simulink model "AC_DC_Converter_SEDC_Motor"  (R2023a)
settings: Solver=VariableStepAuto  StartTime=0.0  StopTime=10  MaxStep=0.001  RelTol=1e-3
libraries: spsThyristorLib x4, spsVoltageMeasurementLib x3, spsSeriesRLCBranchLib x2, simulink x2, dspswit3 x1, spsUniversalBridgeLib x1, spsACVoltageSourceLib x1, sps_lib x1
settings Model: Creator=Mohamed Ezzelrgal  LastModifiedBy=Mohamed Ezzelrgal

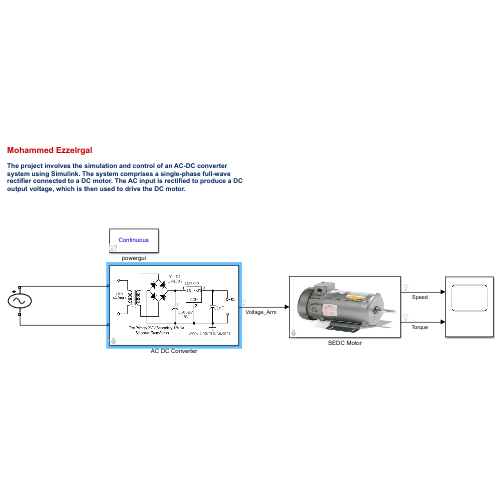
[thumbnail: Simulink's stored preview of the top-level diagram]
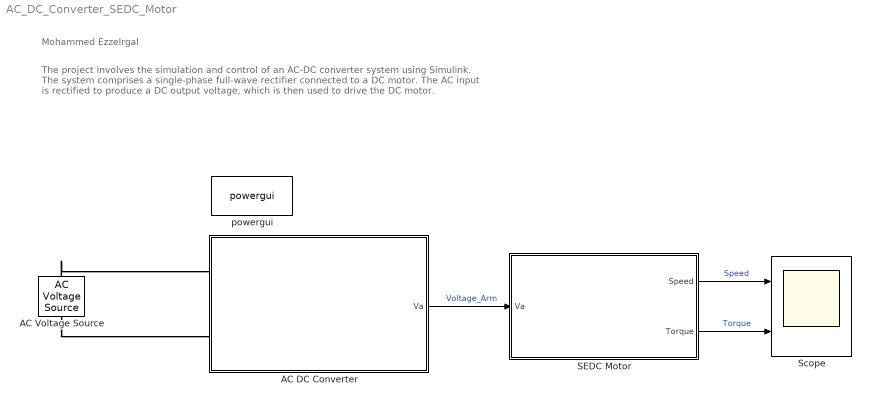
== system AC_DC_Converter_SEDC_Motor ==
  note: Mohammed Ezzelrgal
  note: The project involves the simulation and control of an AC-DC converter system using Simulink. The system comprises a single-phase full-wave rectifier connected to a DC motor. The AC input is rectified to produce a DC output voltage, which is then used to drive the DC motor.
  AC DC Converter : Subsystem  mask{Firing_Angle=20}
      mask prompts: Firing_Angle "Firing Angle"
      mask DialogControl DescGroupVar Prompt: AC-DC Converter
      mask DialogControl DescTextVar Prompt: This conversion process involves changing the polarity of the input AC voltage to produce a unidirectional flow of current in the output DC circuit. AC-DC converters are essential components in various electronic devices and power supplies, allowing them to operate using DC power from an AC power source.
      mask Display: image('acdc.png');
  AC Voltage Source : spsACVoltageSourceLib/AC Voltage Source  Amplitude=sqrt(2)*20  Phase=0  Frequency=50  SampleTime=0  Measurements=None  BusType=swing  Pref=10e3  Qref=0  Qmin=-inf  Qmax=+inf
  SEDC Motor : Subsystem  mask{La=0.1, K_phi=1.6, TL=20, Ra=0.5, J=5, B=0.01}
      mask prompts: K_phi "K Phi"; TL "Torqu Load"
      mask DialogControl DescGroupVar Prompt: SEDC Motor
      mask DialogControl DescTextVar Prompt: Modeling a separately excited DC motor in Simulink involves representing the electrical and mechanical components of the  motor system
      mask Display: image('SEDC.png');
  Scope : Scope  NumInputPorts=2
  powergui : sps_lib/powergui  Priority=1  SimulationMode=Continuous  SampleTime=50e-6  frequency=60  Iterations=50  frequencyindice=50  Pbase=100e6  ErrMax=1e-4  UnitsV=kV  UnitsW=MW  buscounter=0  FunctionMessages=off  echomessages=off  EnableUseOfTLC=off  CurrentSourceSwitches=off  DisableSnubberDevices=off  DisableRonSwitches=off  DisableVfSwitches=off  DisplayEquations=off  AutomaticDiscreteSolvers=off  SolverType=Tustin/Backward Euler (TBE)  Interpol=off  ExternalGateDelay=off  methode=off  Ts=100  x0status=blocks  SPID=on  SwTol=0  HookPort=off  NonlinearTolerance=1e-4  nMaxIteration=100  ContinueOnMaxIteration=off  RestoreLinks=warning  ResistiveCurrentMeasurement=off  Frange=[0:2:500]  Ylog=off  Xlog=on  ShowGrid=off  save=off  variable=ZData  structure=0  ZoomFFT=off  StartTime=0.0  cycles=1  DisplayStyle=1  fundamental=60  FreqAxis=off  MaxFrequency=1000  frequencyindicesteady=1  RmsSteady=1  display=off
  wires:
  SEDC Motor/2(Torque) -> Scope/2  "Torque"
  SEDC Motor/1(Speed) -> Scope/1  "Speed"
  AC DC Converter/1(Va) -> SEDC Motor/1(Va)  "Voltage_Arm"
  connections:
  AC Voltage Source/RConn1 -- AC DC Converter/LConn1
  AC Voltage Source/LConn1 -- AC DC Converter/LConn2

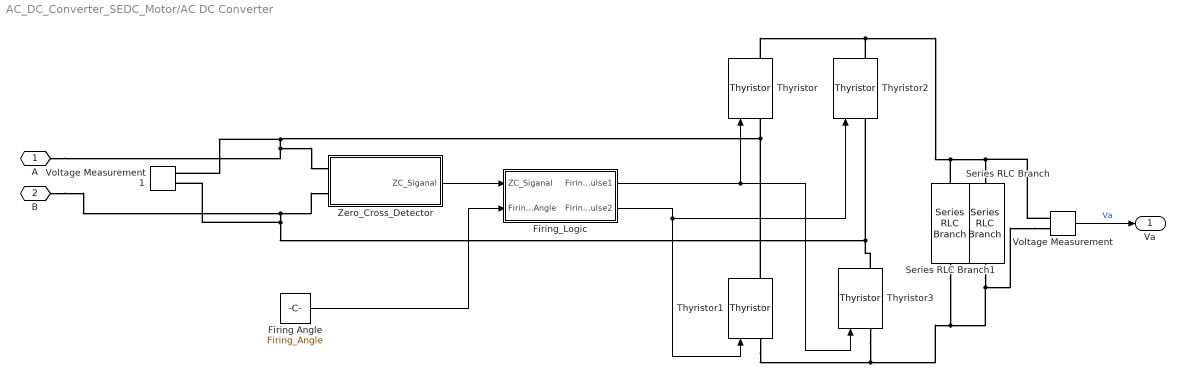
== system AC_DC_Converter_SEDC_Motor/AC DC Converter ==
  Firing Angle : Constant  Value=Firing_Angle
  Firing_Logic : Subsystem
  Series RLC Branch : spsSeriesRLCBranchLib/Series RLC Branch  LConnTagsString=__new0  RConnTagsString=__new0  BranchType=R  Resistance=50  Inductance=1e-3  SetiL0=off  InitialCurrent=0  Capacitance=1e-6  Setx0=off  InitialVoltage=0  Measurements=None
  Series RLC Branch1 : spsSeriesRLCBranchLib/Series RLC Branch  LConnTagsString=__new0  RConnTagsString=__new0  BranchType=C  Resistance=50  Inductance=1e-3  SetiL0=off  InitialCurrent=0  Capacitance=1  Setx0=off  InitialVoltage=0  Measurements=None
  Thyristor{,1..3} (4 alike) : spsThyristorLib/Thyristor  Ron=0.001  Lon=0  Vf=0.8  IC=0  Rs=500  Cs=250e-9  Measurements=on
  Voltage Measurement : spsVoltageMeasurementLib/Voltage Measurement  PhasorSimulation=off  OutputType=Complex  PSBequivalent=0
  Voltage Measurement1 : spsVoltageMeasurementLib/Voltage Measurement  PhasorSimulation=off  OutputType=Complex  PSBequivalent=0
  Zero_Cross_Detector : Subsystem
  A : PMIOPort  Side=Left
  B : PMIOPort  Port=2  Side=Left
  Va : Outport
  wires:
  Firing_Logic/1(Firing_Pulse1) -> Thyristor3/1, Thyristor/1
  Firing_Logic/2(Firing_Pulse2) -> Thyristor2/1, Thyristor1/1
  Zero_Cross_Detector/1(ZC_Siganal) -> Firing_Logic/1(ZC_Siganal)
  Firing Angle/1 -> Firing_Logic/2(Firing_Angle)
  Voltage Measurement/1 -> Va/1  "Va"
  connections:
  Voltage Measurement1/LConn1 -- Thyristor2/LConn1 -- Thyristor3/RConn1 -- B/RConn1 -- Zero_Cross_Detector/LConn2
  Voltage Measurement1/LConn2 -- Thyristor1/RConn1 -- Thyristor/LConn1 -- A/RConn1 -- Zero_Cross_Detector/LConn1
  Thyristor2/RConn1 -- Thyristor/RConn1 -- Series RLC Branch1/LConn1 -- Voltage Measurement/LConn1 -- Series RLC Branch/LConn1
  Voltage Measurement/LConn2 -- Series RLC Branch1/RConn1 -- Thyristor1/LConn1 -- Thyristor3/LConn1 -- Series RLC Branch/RConn1

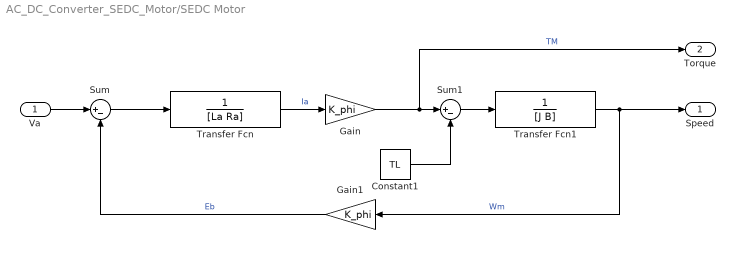
== system AC_DC_Converter_SEDC_Motor/SEDC Motor ==
  Va : Inport
  Constant1 : Constant  Value=TL
  Gain : Gain  Gain=K_phi
  Gain1 : Gain  Gain=K_phi
  Sum : Sum  Inputs=|+-
  Sum1 : Sum  Inputs=|+-
  Transfer Fcn : TransferFcn  Denominator=[La Ra]
  Transfer Fcn1 : TransferFcn  Denominator=[J B]
  Speed : Outport
  Torque : Outport  Port=2
  wires:
  Transfer Fcn/1 -> Gain/1  "Ia"
  Transfer Fcn1/1 -> Speed/1, Gain1/1  "Wm"
  Va/1 -> Sum/1
  Gain1/1 -> Sum/2  "Eb"
  Constant1/1 -> Sum1/2
  Sum/1 -> Transfer Fcn/1
  Gain/1 -> Torque/1, Sum1/1  "TM"
  Sum1/1 -> Transfer Fcn1/1

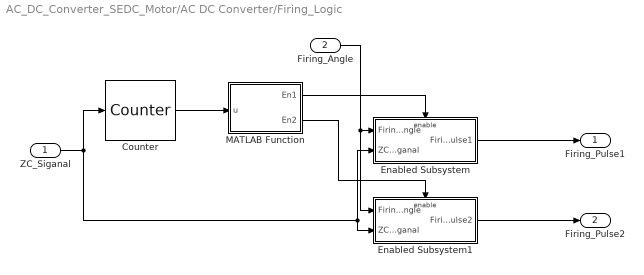
== system AC_DC_Converter_SEDC_Motor/AC DC Converter/Firing_Logic ==
  ZC_Siganal : Inport
  Firing_Angle : Inport  Port=2
  Counter : dspswit3/Counter  Direction=Up  CountEvent=Rising edge  CounterSize=User defined  MaxCount=255  InitialCount=0  Output=Count  HitValue=32  ResetInput=off  SamplesPerFrame=1  Ts=1  CntDtype=double  HitDtype=Logical
  Enabled Subsystem : Subsystem  TreatAsAtomicUnit=on
  Enabled Subsystem1 : Subsystem  TreatAsAtomicUnit=on
  MATLAB Function : MATLAB Function  TreatAsAtomicUnit=on
  Firing_Pulse1 : Outport
  Firing_Pulse2 : Outport  Port=2
  wires:
  ZC_Siganal/1 -> Enabled Subsystem/2(ZC_Siganal), Enabled Subsystem1/2(ZC_Siganal), Counter/1
  Counter/1 -> MATLAB Function/1(u)
  MATLAB Function/1(En1) -> Enabled Subsystem/Enable
  MATLAB Function/2(En2) -> Enabled Subsystem1/Enable
  Firing_Angle/1 -> Enabled Subsystem1/1(Firing_Angle), Enabled Subsystem/1(Firing_Angle)
  Enabled Subsystem/1(Firing_Pulse1) -> Firing_Pulse1/1
  Enabled Subsystem1/1(Firing_Pulse2) -> Firing_Pulse2/1

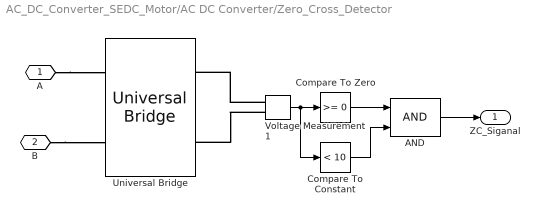
== system AC_DC_Converter_SEDC_Motor/AC DC Converter/Zero_Cross_Detector ==
  AND : Logic  IconShape=distinctive  AllPortsSameDT=off  OutDataTypeStr=boolean
  Compare To Constant : simulink/Logic and Bit Operations/Compare To Constant  relop=<  const=10  OutDataTypeStr=boolean
  Compare To Zero : simulink/Logic and Bit Operations/Compare To Zero  relop=>=  OutDataTypeStr=boolean
  Universal Bridge : spsUniversalBridgeLib/Universal Bridge  Arms=2  SnubberResistance=1e5  SnubberCapacitance=inf  Device=Diodes  Ron=1e-3  Lon=0  ForwardVoltages="[  0  0  ]"  ForwardVoltage=0  GTOparameters=[ 10e-6 , 20e-6 ]  IGBTparameters=[ 1e-6 , 2e-6 ]  Measurements=None  Measurements_2=None  converterType=Rectifier
  Voltage Measurement1 : spsVoltageMeasurementLib/Voltage Measurement  PhasorSimulation=off  OutputType=Complex  PSBequivalent=0
  A : PMIOPort  Side=Left
  B : PMIOPort  Port=2  Side=Left
  ZC_Siganal : Outport
  wires:
  Voltage Measurement1/1 -> Compare To Constant/1, Compare To Zero/1
  Compare To Zero/1 -> AND/1
  Compare To Constant/1 -> AND/2
  AND/1 -> ZC_Siganal/1
  connections:
  B/RConn1 -- Universal Bridge/LConn2
  A/RConn1 -- Universal Bridge/LConn1
  Voltage Measurement1/LConn1 -- Universal Bridge/RConn1
  Voltage Measurement1/LConn2 -- Universal Bridge/RConn2

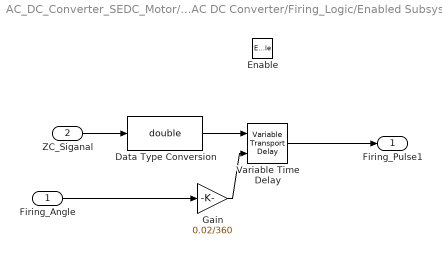
== system AC_DC_Converter_SEDC_Motor/AC DC Converter/Firing_Logic/Enabled Subsystem ==
  Firing_Angle : Inport
  ZC_Siganal : Inport  Port=2
  Enable : EnablePort
  Data Type Conversion : DataTypeConversion  OutDataTypeStr=double  SaturateOnIntegerOverflow=off  RndMeth=Floor
  Gain : Gain  Gain=0.02/360
  Variable Time Delay : VariableTransportDelay  MaximumDelay=10
  Firing_Pulse1 : Outport
  wires:
  ZC_Siganal/1 -> Data Type Conversion/1
  Firing_Angle/1 -> Gain/1
  Gain/1 -> Variable Time Delay/2
  Variable Time Delay/1 -> Firing_Pulse1/1
  Data Type Conversion/1 -> Variable Time Delay/1

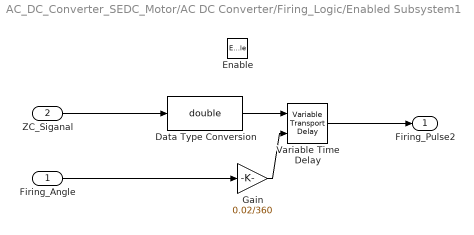
== system AC_DC_Converter_SEDC_Motor/AC DC Converter/Firing_Logic/Enabled Subsystem1 ==
  Firing_Angle : Inport
  ZC_Siganal : Inport  Port=2
  Enable : EnablePort
  Data Type Conversion : DataTypeConversion  OutDataTypeStr=double  SaturateOnIntegerOverflow=off  RndMeth=Floor
  Gain : Gain  Gain=0.02/360
  Variable Time Delay : VariableTransportDelay  MaximumDelay=10
  Firing_Pulse2 : Outport
  wires:
  Data Type Conversion/1 -> Variable Time Delay/1
  Variable Time Delay/1 -> Firing_Pulse2/1
  Gain/1 -> Variable Time Delay/2
  Firing_Angle/1 -> Gain/1
  ZC_Siganal/1 -> Data Type Conversion/1

== matlab function AC_DC_Converter_SEDC_Motor/AC DC Converter/Firing_Logic/MATLAB Function ==
  data: u input; En1 output; En2 output
function [En1, En2] = fcn(u)
En1 = 0 ;
En2 = 0 ;

if mod(u,2) == 0
  En1 = 1 ;
  En2 = 0 ;

end

if mod(u,2) == 1
  En1 = 0 ;
  En2 = 1 ;

end
